simulink model "heat_exchange"  (R2023b)
settings: Solver=VariableStepAuto  StartTime=0.0  StopTime=10.0  RelTol=1e-3
values from neighbouring files (symbols this model uses):
  a_b = 6*(1-eps_bed)/(r_p*2)    (= 200)    [DRI_furnace_loader.m]
  dz = ones(1, n_furnace+1)* (h_furnace/(n_furnace-1))    [DRI_furnace_loader.m]
  n_furnace = 75    [DRI_furnace_loader.m]
  T_ginit = interp1([1:1:length(T_ginit)],T_ginit, linspace(1,length(T_ginit),n_furnace))    [DRI_furnace_loader.m]    (also in inital_conditions.m = out.T_g.data(end,2:end); initcond.mat = [1196.65645819 1175.51158545 1159.95869756 1147.6627975 1137; initcond_H2.mat = [1206.04002008 1196.92003246 1187.72467669 1178.52571193 116; initcond_NG.mat = [1059.94701026 1050.97990802 1047.95611626 1045.20600654 104)
  T_sinit = interp1([1:1:length(T_sinit)],T_sinit, linspace(1,length(T_sinit),n_furnace))    [DRI_furnace_loader.m]    (also in inital_conditions.m = out.T_s.data(end,1:end-1); initcond.mat = [1154.84636481 1150.12425371 1141.69055851 1133.58197665 112; initcond_H2.mat = [1198.21532505 1188.90892541 1179.58573027 1170.31082456 116; initcond_NG.mat = [1055.14966191 1048.70059171 1045.82868823 1043.13322913 104)
settings Model: Creator=jimmonen  LastModifiedBy=jimmonen

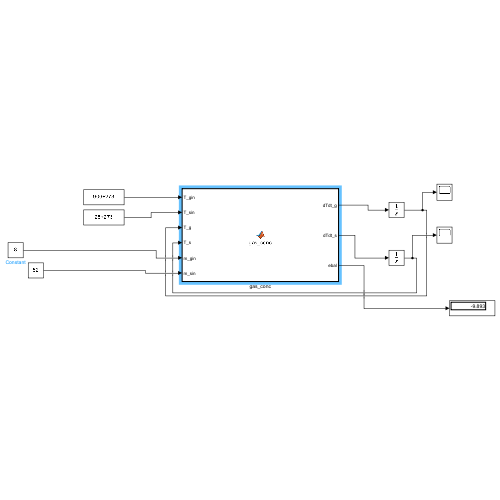
[thumbnail: Simulink's stored preview of the top-level diagram]
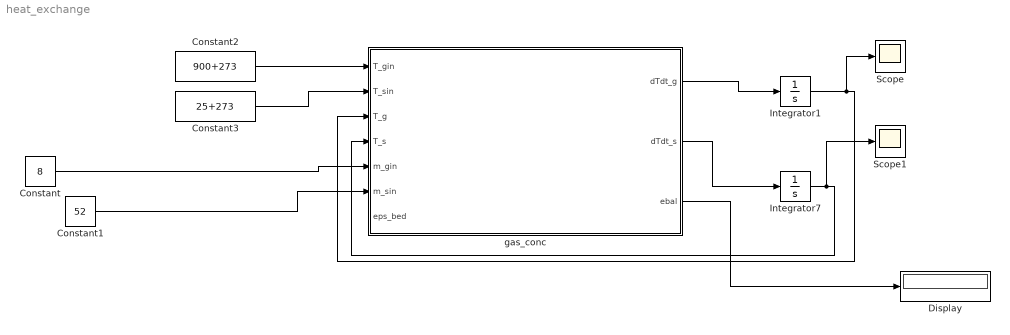
== system heat_exchange ==
  Constant : Constant  Value=8
  Constant1 : Constant  Value=52
  Constant2 : Constant  Value=900+273
  Constant3 : Constant  Value=25+273
  Display : Display
  Integrator1 : Integrator  InitialCondition=T_ginit
  Integrator7 : Integrator  InitialCondition=T_sinit
  Scope : Scope
  Scope1 : Scope
  gas_conc : MATLAB Function  TreatAsAtomicUnit=on
  wires:
  gas_conc/2(dTdt_s) -> Integrator7/1
  gas_conc/1(dTdt_g) -> Integrator1/1
  Integrator1/1 -> Scope/1, gas_conc/3(T_g)
  Constant/1 -> gas_conc/5(m_gin)
  Constant1/1 -> gas_conc/6(m_sin)
  Integrator7/1 -> Scope1/1, gas_conc/4(T_s)
  Constant2/1 -> gas_conc/1(T_gin)
  Constant3/1 -> gas_conc/2(T_sin)
  gas_conc/3(ebal) -> Display/1

== matlab function heat_exchange/gas_conc ==
  data: T_gin input; T_sin input; T_g input; T_s input; m_gin input; dTdt_g output; m_sin input; dTdt_s output; dz parameter; n_furnace parameter; a_b parameter; ebal output; eps_bed input
function [dTdt_g, dTdt_s, ebal] = gas_conc(T_gin, T_sin, T_g, T_s, m_gin, m_sin, dz, n_furnace, a_b, eps_bed)

u_g = 20;
u_s = 0.0005;

method = "UPWIND";

Cp_s = 600;
Cp_g = 10000;

rho_b = 4750;
rho_g = 0.027;

h_sg = 25;

dTdt_s = zeros(size(T_s));
dTdt_g = zeros(size(T_g));

%F_T_s = -flip(Flux_Limiter(flip(T_s), T_sin, u_s, dz, method));

F_T_s = -Flux_Limiter(T_s, T_sin, u_s, dz, method);
F_T_g = -Flux_Limiter(T_g, T_gin, u_g, dz, method);

a_1 = 1;
a_2 = 2;

for i = 1:n_furnace
    
    %added 0.6!!!!
    dTdt_s(i) = F_T_s(i) + ((a_b*h_sg)/(rho_b*Cp_s)*(1-eps_bed))*(T_g(i)-T_s(i));
    dTdt_g(i) = F_T_g(i) + ((a_b*h_sg)/(rho_g*Cp_g*eps_bed)*(T_s(i)-T_g(i)));
    
end

%energy_in = m_gin*Cp_g*T_gin + m_sin*Cp_s*T_sin; 
%energy_out = m_gin*Cp_g*T_g(end) + m_sin*Cp_s*T_s(1); 


energy_in = m_gin*Cp_g*T_gin + m_sin*Cp_s*T_sin; 
energy_out = m_gin*Cp_g*T_g(end) + m_sin*Cp_s*T_s(end); 

ebal = (energy_in - energy_out)/1e6;
